simulink model "aircraft_arch"  (R2024a)
settings: Solver=FixedStepAuto  StartTime=0.0  StopTime=100.0  FixedStep=0.1  RelTol=1e-3
settings Model: Creator=amir  LastModifiedBy=amir
settings ConfigComp: CovEnable=on  RecordCoverage=on  CovEnableCumulative=off  CovModelRefEnable=on

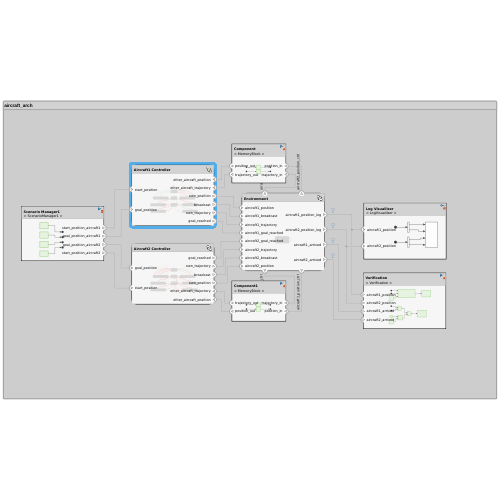
[thumbnail: Simulink's stored preview of the top-level diagram]
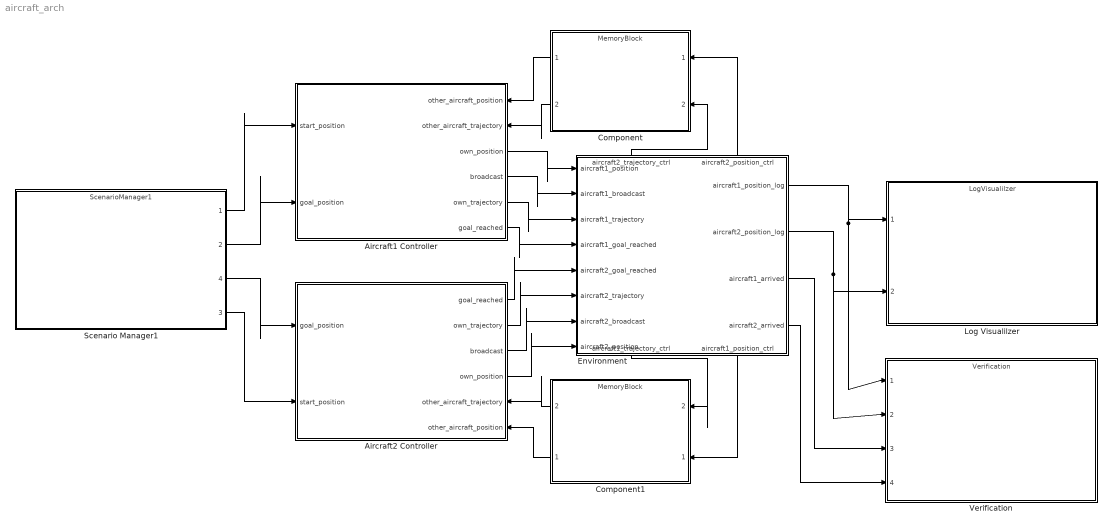
== system aircraft_arch ==
  Aircraft1 Controller : Stateflow chart  TreatAsAtomicUnit=on
      settings: PortSchema="{\"entries\":[{\"content\":{\"headerSize\":26,\"margin\":15,\"minimumSpacing\":25,\"sides\":[{\"content\":{\"connectorIds\":[\"In3\",\"In4\"]},\"type\":\"ConnectorPlacement.EquallySpacedRectSide\",\"uuid\":\"1f55804f-7089-4bd3-b638-e4b9c8b42ca4\"},{\"content\":{\"connectorIds\":[\"In1\",\"In2\",\"Out1\",\"Out2\",\"Out3\",\"Out4\"],\"side\":\"RIGHT\"},\"type\":\"ConnectorPlacement.EquallySpacedRectSide\",\"uuid\":\"b3c2471c-8380-46f0-98ab-243070185840\"},{\"content\":{\"side\":\"TOP\"},\"type\":\"ConnectorPlacement.EquallySpacedRectSide\",\"uuid\":\"f84a374d-020b-4849-aef2-6fb46c6d88bf\"}]},\"type\":\"ConnectorPlacement.EquallySpacedConnector\",\"uuid\":\"5317393d-ba95-4fee-8ac3-0dbadcfc5ad7\"}],\"packageUris\":[\"http://schema.mathworks.com/mf0/Connector/R2020b\"],\"version\":\"1.0\"}"
  Aircraft2 Controller : Stateflow chart  TreatAsAtomicUnit=on
      settings: PortSchema="{\"entries\":[{\"content\":{\"headerSize\":26,\"margin\":15,\"minimumSpacing\":25,\"sides\":[{\"content\":{\"connectorIds\":[\"In4\",\"In3\"]},\"type\":\"ConnectorPlacement.EquallySpacedRectSide\",\"uuid\":\"1f55804f-7089-4bd3-b638-e4b9c8b42ca4\"},{\"content\":{\"connectorIds\":[\"Out4\",\"Out3\",\"Out2\",\"Out1\",\"In1\",\"In2\"],\"side\":\"RIGHT\"},\"type\":\"ConnectorPlacement.EquallySpacedRectSide\",\"uuid\":\"b3c2471c-8380-46f0-98ab-243070185840\"},{\"content\":{\"side\":\"TOP\"},\"type\":\"ConnectorPlacement.EquallySpacedRectSide\",\"uuid\":\"f84a374d-020b-4849-aef2-6fb46c6d88bf\"}]},\"type\":\"ConnectorPlacement.EquallySpacedConnector\",\"uuid\":\"5317393d-ba95-4fee-8ac3-0dbadcfc5ad7\"}],\"packageUris\":[\"http://schema.mathworks.com/mf0/Connector/R2020b\"],\"version\":\"1.0\"}"
  Component : ModelReference  ModelNameDialog=MemoryBlock.slx  SimulationMode=Normal  ModelReferenceVersion=1.4
      settings: PortSchema="{\"entries\":[{\"content\":{\"headerSize\":38,\"margin\":15,\"minimumSpacing\":25,\"sides\":[{\"content\":{\"connectorIds\":[\"Out1\",\"Out2\"]},\"type\":\"ConnectorPlacement.EquallySpacedRectSide\",\"uuid\":\"1f55804f-7089-4bd3-b638-e4b9c8b42ca4\"},{\"content\":{\"connectorIds\":[\"In1\",\"In2\"],\"side\":\"RIGHT\"},\"type\":\"ConnectorPlacement.EquallySpacedRectSide\",\"uuid\":\"b3c2471c-8380-46f0-98ab-243070185840\"},{\"content\":{\"side\":\"TOP\"},\"type\":\"ConnectorPlacement.EquallySpacedRectSide\",\"uuid\":\"f84a374d-020b-4849-aef2-6fb46c6d88bf\"},{\"content\":{\"side\":\"BOTTOM\"},\"type\":\"ConnectorPlacement.EquallySpacedRectSide\",\"uuid\":\"1d177eb2-3e23-41ae-8748-2ec0886adf75\"}]},\"type\":\"ConnectorPlacement.EquallySpacedConnector\",\"uuid\":\"5317393d-ba95-4fee-8ac3-0dbadcfc5ad7\"}],\"packageUris\":[\"http://schema.mathworks.com/mf0/Connector/R2020b\"],\"version\":\"1.0\"}"
  Component1 : ModelReference  ModelNameDialog=MemoryBlock  SimulationMode=Normal  ModelReferenceVersion=1.4
      settings: PortSchema="{\"entries\":[{\"content\":{\"headerSize\":38,\"margin\":15,\"minimumSpacing\":25,\"sides\":[{\"content\":{\"connectorIds\":[\"Out2\",\"Out1\"]},\"type\":\"ConnectorPlacement.EquallySpacedRectSide\",\"uuid\":\"1f55804f-7089-4bd3-b638-e4b9c8b42ca4\"},{\"content\":{\"connectorIds\":[\"In2\",\"In1\"],\"side\":\"RIGHT\"},\"type\":\"ConnectorPlacement.EquallySpacedRectSide\",\"uuid\":\"b3c2471c-8380-46f0-98ab-243070185840\"},{\"content\":{\"side\":\"TOP\"},\"type\":\"ConnectorPlacement.EquallySpacedRectSide\",\"uuid\":\"f84a374d-020b-4849-aef2-6fb46c6d88bf\"},{\"content\":{\"side\":\"BOTTOM\"},\"type\":\"ConnectorPlacement.EquallySpacedRectSide\",\"uuid\":\"1d177eb2-3e23-41ae-8748-2ec0886adf75\"}]},\"type\":\"ConnectorPlacement.EquallySpacedConnector\",\"uuid\":\"5317393d-ba95-4fee-8ac3-0dbadcfc5ad7\"}],\"packageUris\":[\"http://schema.mathworks.com/mf0/Connector/R2020b\"],\"version\":\"1.0\"}"
  Environment : Stateflow chart  TreatAsAtomicUnit=on
      settings: PortSchema="{\"entries\":[{\"content\":{\"headerSize\":26,\"margin\":15,\"minimumSpacing\":25,\"sides\":[{\"content\":{\"connectorIds\":[\"In1\",\"In2\",\"In3\",\"In4\",\"In5\",\"In6\",\"In7\",\"In8\"]},\"type\":\"ConnectorPlacement.EquallySpacedRectSide\",\"uuid\":\"1f55804f-7089-4bd3-b638-e4b9c8b42ca4\"},{\"content\":{\"connectorIds\":[\"Out1\",\"Out4\",\"Out7\",\"Out8\"],\"side\":\"RIGHT\"},\"type\":\"ConnectorPlacement.EquallySpacedRectSide\",\"uuid\":\"b3c2471c-8380-46f0-98ab-243070185840\"},{\"content\":{\"connectorIds\":[\"Out3\",\"Out5\"],\"side\":\"TOP\"},\"type\":\"ConnectorPlacement.EquallySpacedRectSide\",\"uuid\":\"f84a374d-020b-4849-aef2-6fb46c6d88bf\"},{\"content\":{\"connectorIds\":[\"Out2\",\"Out6\"],\"side\":\"BOTTOM\"},\"type\":\"ConnectorPlacement.EquallySpacedRectSide\",\"uuid\":\"852cc804-b545-4d00-b17f-3ae2fc6b003e\"}]},\"type\":\"ConnectorPlacement.EquallySpacedConnector\",\"uuid\":\"5317393d-ba95-4fee-8ac3-0dbadcfc5ad7\"}],\"packageUris\":[\"http://schema.mathworks.com/mf0/Connector/R2020b\"],\"version\":\"1.0\"}"
  Log Visualilzer : ModelReference  ModelNameDialog=LogVisualilzer  SimulationMode=Normal  ModelReferenceVersion=1.7
      settings: PortSchema="{\"entries\":[{\"content\":{\"headerSize\":38,\"margin\":15,\"minimumSpacing\":25,\"sides\":[{\"content\":{\"connectorIds\":[\"In1\",\"In2\"]},\"type\":\"ConnectorPlacement.EquallySpacedRectSide\",\"uuid\":\"1f55804f-7089-4bd3-b638-e4b9c8b42ca4\"},{\"content\":{\"side\":\"RIGHT\"},\"type\":\"ConnectorPlacement.EquallySpacedRectSide\",\"uuid\":\"b3c2471c-8380-46f0-98ab-243070185840\"},{\"content\":{\"side\":\"TOP\"},\"type\":\"ConnectorPlacement.EquallySpacedRectSide\",\"uuid\":\"f84a374d-020b-4849-aef2-6fb46c6d88bf\"}]},\"type\":\"ConnectorPlacement.EquallySpacedConnector\",\"uuid\":\"5317393d-ba95-4fee-8ac3-0dbadcfc5ad7\"}],\"packageUris\":[\"http://schema.mathworks.com/mf0/Connector/R2020b\"],\"version\":\"1.0\"}"
  Scenario Manager1 : ModelReference  ModelNameDialog=ScenarioManager1.slx  SimulationMode=Normal  ModelReferenceVersion=1.20
      settings: PortSchema="{\"entries\":[{\"content\":{\"headerSize\":38,\"margin\":15,\"minimumSpacing\":25,\"sides\":[{\"content\":{},\"type\":\"ConnectorPlacement.EquallySpacedRectSide\",\"uuid\":\"1f55804f-7089-4bd3-b638-e4b9c8b42ca4\"},{\"content\":{\"connectorIds\":[\"Out1\",\"Out2\",\"Out4\",\"Out3\"],\"side\":\"RIGHT\"},\"type\":\"ConnectorPlacement.EquallySpacedRectSide\",\"uuid\":\"b3c2471c-8380-46f0-98ab-243070185840\"},{\"content\":{\"side\":\"TOP\"},\"type\":\"ConnectorPlacement.EquallySpacedRectSide\",\"uuid\":\"f84a374d-020b-4849-aef2-6fb46c6d88bf\"}]},\"type\":\"ConnectorPlacement.EquallySpacedConnector\",\"uuid\":\"5317393d-ba95-4fee-8ac3-0dbadcfc5ad7\"}],\"packageUris\":[\"http://schema.mathworks.com/mf0/Connector/R2020b\"],\"version\":\"1.0\"}"
  Verification : ModelReference  ModelNameDialog=Verification  SimulationMode=Normal  ModelReferenceVersion=1.8
      settings: PortSchema="{\"entries\":[{\"content\":{\"headerSize\":38,\"margin\":15,\"minimumSpacing\":25,\"sides\":[{\"content\":{\"connectorIds\":[\"In1\",\"In2\",\"In3\",\"In4\"]},\"type\":\"ConnectorPlacement.EquallySpacedRectSide\",\"uuid\":\"10c170e3-5d79-4eda-90c6-d87a95188a44\"},{\"content\":{\"side\":\"RIGHT\"},\"type\":\"ConnectorPlacement.EquallySpacedRectSide\",\"uuid\":\"ea2fd0a6-7ce8-495f-a83e-fe6cf76b2057\"},{\"content\":{\"side\":\"TOP\"},\"type\":\"ConnectorPlacement.EquallySpacedRectSide\",\"uuid\":\"87f50319-688b-4f7c-b51e-7381fe44f37b\"}]},\"type\":\"ConnectorPlacement.EquallySpacedConnector\",\"uuid\":\"e134149c-ef09-4213-a414-03764e4b3756\"}],\"packageUris\":[\"http://schema.mathworks.com/mf0/Connector/R2020b\"],\"version\":\"1.0\"}"
  wires:
  Scenario Manager1/2 -> Aircraft1 Controller/4(goal_position)
  Scenario Manager1/1 -> Aircraft1 Controller/3(start_position)
  Scenario Manager1/4 -> Aircraft2 Controller/4(goal_position)
  Scenario Manager1/3 -> Aircraft2 Controller/3(start_position)
  Aircraft1 Controller/1(own_position) -> Environment/1(aircraft1_position)
  Aircraft2 Controller/1(own_position) -> Environment/8(aircraft2_position)
  Aircraft2 Controller/2(broadcast) -> Environment/7(aircraft2_broadcast)
  Aircraft1 Controller/2(broadcast) -> Environment/2(aircraft1_broadcast)
  Environment/5(aircraft2_position_ctrl) -> Component/1
  Component/1 -> Aircraft1 Controller/1(other_aircraft_position)
  Component1/1 -> Aircraft2 Controller/2(other_aircraft_position)
  Aircraft1 Controller/3(own_trajectory) -> Environment/3(aircraft1_trajectory)
  Aircraft1 Controller/4(goal_reached) -> Environment/4(aircraft1_goal_reached)
  Environment/6(aircraft1_position_ctrl) -> Component1/1
  Aircraft2 Controller/3(own_trajectory) -> Environment/6(aircraft2_trajectory)
  Aircraft2 Controller/4(goal_reached) -> Environment/5(aircraft2_goal_reached)
  Environment/3(aircraft2_trajectory_ctrl) -> Component/2
  Component/2 -> Aircraft1 Controller/2(other_aircraft_trajectory)
  Environment/2(aircraft1_trajectory_ctrl) -> Component1/2
  Component1/2 -> Aircraft2 Controller/1(other_aircraft_trajectory)
  Environment/7(aircraft1_arrived) -> Verification/3
  Environment/1(aircraft1_position_log) -> Log Visualilzer/1, Verification/1
  Environment/8(aircraft2_arrived) -> Verification/4
  Environment/4(aircraft2_position_log) -> Log Visualilzer/2, Verification/2

== stateflow chart aircraft_arch/Aircraft2 Controller ==
  settings: updateMethod=CONTINUOUS
  state Idle
    during:
    own_position_dot(1) = 0;
    own_position_dot(2) = 0;
    broadcast = true;
  state CombsDelay
    during:
    own_position_dot(1) = 0;
    own_position_dot(2) = 0;
    broadcast = false;
  state VerticalMovement
    during:
    own_position_dot(2) = sign(goal_position(2) - own_position(2));
  state HorizontalMovement
    during:
    own_position_dot(1) = sign(goal_position(1) - own_position(1));
  state CorrectionManager
    during:
    own_position_dot(1) = 0;
    own_position_dot(2) = 0;
    broadcast = true;
  state HorizontalHeadOn_Side_CollisionAvoidance_VerticalMovement
    during:
    own_position_dot(1) = own_trajectory(2);
    own_position_dot(2) = -own_trajectory(1);
  state VerticalHeadOn_CollisionAvoidance_HorizontalMovement
    during:
    own_position_dot(1) = own_trajectory(2);
    own_position_dot(2) = -own_trajectory(1);
  state VerticalHeadOnCollisionAvoidanc_VerticalMovement
    during:
    own_position_dot(1) = own_trajectory(1);
    own_position_dot(2) = own_trajectory(2);
  state HeadButt_CollisionAvoidance
    during:
    own_position_dot(1) = -other_aircraft_trajectory(1);
    own_position_dot(2) = -other_aircraft_trajectory(2);
  (default) -> Idle : {own_position = start_position;
      | broadcast = true;
      | own_trajectory = [0, 0];
      | head_on_correction_step = 0;
      | vertical_trajectory=false;}
  VerticalMovement -> Idle [order 1] : [(abs(own_position(2) - round(own_position(2))) <= 0.01) && (abs(own_position(1) - goal_position(1)) > 0.01)]
      | {own_trajectory(1) = sign(goal_position(1) - own_position(1)); own_trajectory(2) = 0; vertical_trajectory = false;}
  HorizontalMovement -> Idle [order 1] : [(abs(own_position(1) - round(own_position(1))) <= 0.01) && (abs(own_position(1) - goal_position(1)) > 0.01)]
      | {own_trajectory(1) = sign(goal_position(1) - own_position(1)); own_trajectory(2) = 0;}
  HorizontalMovement -> Idle [order 2] : [(abs(own_position(1) - round(own_position(1))) <= 0.01) && (abs(own_position(2) - goal_position(2)) > 0.01)]
      | {own_trajectory(1) = 0; own_trajectory(2) = sign(goal_position(2) - own_position(2));}
  VerticalMovement -> Idle [order 2] : [(abs(own_position(2) - round(own_position(2))) <= 0.01) && (abs(own_position(2) - goal_position(2)) > 0.01)]
      | {own_trajectory(1) = 0; own_trajectory(2) = sign(goal_position(2) - own_position(2)); vertical_trajectory = false;}
  VerticalMovement -> Idle [order 3] : [(abs(own_position(1) - round(own_position(1))) <= 0.01) && (abs(own_position(2) - round(own_position(2))) <= 0.01)]
      | {goal_reached = true; vertical_trajectory = false;}
  HorizontalMovement -> Idle [order 3] : [(abs(own_position(1) - round(own_position(1))) <= 0.01) && (abs(own_position(2) - round(own_position(2))) <= 0.01)]
      | {goal_reached = true;}
  Idle -> CombsDelay : [(abs(own_position(1) - goal_position(1)) > 0.01) || (abs(own_position(2) - goal_position(2)) > 0.01)]
  CombsDelay -> HorizontalMovement [order 4] : [(abs(own_position(1) - goal_position(1)) > 0.01) && ~vertical_trajectory]
  CombsDelay -> VerticalMovement [order 5] : [(abs(own_position(2) - goal_position(2)) > 0.01) || vertical_trajectory]
  CombsDelay -> (junction 360) [order 1] : [(all(round(own_position) + own_trajectory == round(other_aircraft_position) + other_aircraft_trajectory) || ...
      |  all(round(own_position) + 0.5 * own_trajectory == round(other_aircraft_position) + 0.5 * other_aircraft_trajectory)) && ...
      |  (all(abs(round(own_trajectory - other_aircraft_trajectory)) == [2, 0]) || ...
      |  all(abs(round(own_trajectory - other_aircraft_trajectory)) == [1, 1]))]
  CombsDelay -> VerticalHeadOn_CollisionAvoidance_HorizontalMovement [order 2] : [(all(round(own_position) + own_trajectory == round(other_aircraft_position) + other_aircraft_trajectory) || ...
      |  all(round(own_position) + 0.5 * own_trajectory == round(other_aircraft_position) + 0.5 * other_aircraft_trajectory)) && ...
      |  all(abs(round(own_trajectory - other_aircraft_trajectory)) == [0, 2])]
      | {head_on_correction_step = abs(round(own_position(2)) - round(other_aircraft_position(2)));}
  CorrectionManager -> CombsDelay [order 2]
  CombsDelay -> (junction 351) [order 3] : [all(round(own_position) + own_trajectory == round(other_aircraft_position))]
  (junction 360) -> HorizontalHeadOn_Side_CollisionAvoidance_VerticalMovement [order 1] : [abs(round(own_trajectory)) == [0, 1]]
      | {vertical_trajectory = true;}
  (junction 360) -> HorizontalHeadOn_Side_CollisionAvoidance_VerticalMovement [order 2]
  VerticalHeadOn_CollisionAvoidance_HorizontalMovement -> CorrectionManager : [(abs(own_position(1) - round(own_position(1))) <= 0.01)]
  HorizontalHeadOn_Side_CollisionAvoidance_VerticalMovement -> CorrectionManager : [(~vertical_trajectory && abs(own_position(2) - round(own_position(2))) <= 0.01) || ...
      |  (vertical_trajectory && abs(own_position(1) - round(own_position(1))) <= 0.01)]
  CorrectionManager -> VerticalHeadOnCollisionAvoidanc_VerticalMovement [order 1] : [head_on_correction_step ~= 0]
  VerticalHeadOnCollisionAvoidanc_VerticalMovement -> CorrectionManager : [(abs(own_position(2) - round(own_position(2))) <= 0.01)]
      | {head_on_correction_step = head_on_correction_step - 1}
  HeadButt_CollisionAvoidance -> CorrectionManager : [(~vertical_trajectory && abs(own_position(2) - round(own_position(2))) <= 0.01) || ...
      |  (vertical_trajectory && abs(own_position(1) - round(own_position(1))) <= 0.01)]
  (junction 351) -> HeadButt_CollisionAvoidance [order 1] : [abs(round(own_trajectory)) == [0, 1]]
      | {vertical_trajectory = true;}
  (junction 351) -> HeadButt_CollisionAvoidance [order 2]
  data: other_aircraft_trajectory input size=[1, 2]; other_aircraft_position input size=[1, 2]; start_position input size=[1, 2]; goal_position input size=[1, 2]; own_position output size=[1, 2]; broadcast output boolean; own_trajectory output size=[1, 2]; goal_reached output boolean; head_on_correction_step local; vertical_trajectory local boolean
  data own_position settings: updateMethod=SF_CONTINUOUS_TIME_DATA
  data own_trajectory settings: updateMethod=SF_CONTINUOUS_TIME_DATA

== stateflow chart aircraft_arch/Environment ==
  settings: updateMethod=CONTINUOUS
  state LogPass
    during:
    aircraft1_position_log = aircraft1_position;
    aircraft2_position_log = aircraft2_position;
    aircraft1_arrived = aircraft1_goal_reached;
    aircraft2_arrived = aircraft2_goal_reached;
  (default) -> LogPass : {aircraft1_position_log = aircraft1_position;
      | aircraft1_position_ctrl = [10000, 10000];
      | aircraft1_trajectory_ctrl = [0, 0];
      | aircraft2_position_log = aircraft2_position;
      | aircraft2_position_ctrl = [10000, 10000];
      | aircraft2_trajectory_ctrl = [0, 0];}
  LogPass -> LogPass [order 2] : [aircraft1_broadcast && aircraft2_broadcast && ...
      |  (aircraft1_goal_reached || aircraft2_goal_reached || ...
      |   (abs(round(aircraft1_position(1)) - round(aircraft2_position(1))) > 2) || ...
      |   (abs(round(aircraft1_position(2)) - round(aircraft2_position(2))) > 2))]
      | {aircraft1_position_ctrl   = [10000, 10000];
      |  aircraft1_trajectory_ctrl = [0, 0];
      |  aircraft2_position_ctrl   = [10000, 10000];
      |  aircraft2_trajectory_ctrl = [0, 0];}
  LogPass -> LogPass [order 1] : [aircraft1_broadcast && aircraft2_broadcast && ...
      |  ~aircraft1_goal_reached && ~aircraft2_goal_reached && ...
      |  (abs(round(aircraft1_position(1)) - round(aircraft2_position(1))) <= 2) && ...
      |  (abs(round(aircraft1_position(2)) - round(aircraft2_position(2))) <= 2)]
      | {aircraft1_position_log = aircraft1_position;
      |  aircraft1_position_ctrl = aircraft1_position;
      |  aircraft1_trajectory_ctrl = aircraft1_trajectory;
      |  aircraft2_position_log = aircraft2_position;
      |  aircraft2_position_ctrl = aircraft2_position;
      |  aircraft2_trajectory_ctrl = aircraft2_trajectory;}
  data: aircraft1_position input size=[1, 2]; aircraft1_broadcast input boolean; aircraft1_trajectory input size=[1, 2]; aircraft1_goal_reached input boolean; aircraft2_goal_reached input boolean; aircraft2_trajectory input size=[1, 2]; aircraft2_broadcast input boolean; aircraft2_position input size=[1, 2]; aircraft1_position_log output size=[1, 2]; aircraft1_trajectory_ctrl output; aircraft2_trajectory_ctrl output; aircraft2_position_log output size=[1, 2]; aircraft2_position_ctrl output size=[1, 2]; aircraft1_position_ctrl output size=[1, 2]; aircraft1_arrived output boolean; aircraft2_arrived output boolean

== stateflow chart aircraft_arch/Aircraft1 Controller ==
  settings: updateMethod=CONTINUOUS
  state Idle
    during:
    own_position_dot(1) = 0;
    own_position_dot(2) = 0;
    broadcast = true;
  state CombsDelay
    during:
    own_position_dot(1) = 0;
    own_position_dot(2) = 0;
    broadcast = false;
  state VerticalMovement
    during:
    own_position_dot(2) = sign(goal_position(2) - own_position(2));
  state HorizontalMovement
    during:
    own_position_dot(1) = sign(goal_position(1) - own_position(1));
  state CorrectionManager
    during:
    own_position_dot(1) = 0;
    own_position_dot(2) = 0;
    broadcast = true;
  state HorizontalHeadOn_Side_CollisionAvoidance_VerticalMovement
    during:
    own_position_dot(1) = own_trajectory(2);
    own_position_dot(2) = -own_trajectory(1);
  state VerticalHeadOn_CollisionAvoidance_HorizontalMovement
    during:
    own_position_dot(1) = own_trajectory(2);
    own_position_dot(2) = -own_trajectory(1);
  state VerticalHeadOnCollisionAvoidanc_VerticalMovement
    during:
    own_position_dot(1) = own_trajectory(1);
    own_position_dot(2) = own_trajectory(2);
  state HeadButt_CollisionAvoidance
    during:
    own_position_dot(1) = -other_aircraft_trajectory(1);
    own_position_dot(2) = -other_aircraft_trajectory(2);
  (default) -> Idle : {own_position = start_position;
      | broadcast = true;
      | own_trajectory = [0, 0];
      | head_on_correction_step = 0;
      | vertical_trajectory=false;}
  VerticalMovement -> Idle [order 1] : [(abs(own_position(2) - round(own_position(2))) <= 0.01) && (abs(own_position(1) - goal_position(1)) > 0.01)]
      | {own_trajectory(1) = sign(goal_position(1) - own_position(1)); own_trajectory(2) = 0; vertical_trajectory = false;}
  HorizontalMovement -> Idle [order 1] : [(abs(own_position(1) - round(own_position(1))) <= 0.01) && (abs(own_position(1) - goal_position(1)) > 0.01)]
      | {own_trajectory(1) = sign(goal_position(1) - own_position(1)); own_trajectory(2) = 0;}
  HorizontalMovement -> Idle [order 2] : [(abs(own_position(1) - round(own_position(1))) <= 0.01) && (abs(own_position(2) - goal_position(2)) > 0.01)]
      | {own_trajectory(1) = 0; own_trajectory(2) = sign(goal_position(2) - own_position(2));}
  VerticalMovement -> Idle [order 2] : [(abs(own_position(2) - round(own_position(2))) <= 0.01) && (abs(own_position(2) - goal_position(2)) > 0.01)]
      | {own_trajectory(1) = 0; own_trajectory(2) = sign(goal_position(2) - own_position(2)); vertical_trajectory = false;}
  VerticalMovement -> Idle [order 3] : [(abs(own_position(1) - round(own_position(1))) <= 0.01) && (abs(own_position(2) - round(own_position(2))) <= 0.01)]
      | {goal_reached = true; vertical_trajectory = false;}
  HorizontalMovement -> Idle [order 3] : [(abs(own_position(1) - round(own_position(1))) <= 0.01) && (abs(own_position(2) - round(own_position(2))) <= 0.01)]
      | {goal_reached = true;}
  Idle -> CombsDelay : [(abs(own_position(1) - goal_position(1)) > 0.01) || (abs(own_position(2) - goal_position(2)) > 0.01)]
  CombsDelay -> HorizontalMovement [order 4] : [(abs(own_position(1) - goal_position(1)) > 0.01) && ~vertical_trajectory]
  CombsDelay -> VerticalMovement [order 5] : [(abs(own_position(2) - goal_position(2)) > 0.01) || vertical_trajectory]
  CombsDelay -> (junction 99) [order 1] : [(all(round(own_position) + own_trajectory == round(other_aircraft_position) + other_aircraft_trajectory) || ...
      |  all(round(own_position) + 0.5 * own_trajectory == round(other_aircraft_position) + 0.5 * other_aircraft_trajectory)) && ...
      |  (all(abs(round(own_trajectory - other_aircraft_trajectory)) == [2, 0]) || ...
      |  all(abs(round(own_trajectory - other_aircraft_trajectory)) == [1, 1]))]
  CombsDelay -> VerticalHeadOn_CollisionAvoidance_HorizontalMovement [order 2] : [(all(round(own_position) + own_trajectory == round(other_aircraft_position) + other_aircraft_trajectory) || ...
      |  all(round(own_position) + 0.5 * own_trajectory == round(other_aircraft_position) + 0.5 * other_aircraft_trajectory)) && ...
      |  all(abs(round(own_trajectory - other_aircraft_trajectory)) == [0, 2])]
      | {head_on_correction_step = abs(round(own_position(2)) - round(other_aircraft_position(2)));}
  CorrectionManager -> CombsDelay [order 2]
  CombsDelay -> (junction 125) [order 3] : [all(round(own_position) + own_trajectory == round(other_aircraft_position))]
  (junction 99) -> HorizontalHeadOn_Side_CollisionAvoidance_VerticalMovement [order 1] : [abs(round(own_trajectory)) == [0, 1]]
      | {vertical_trajectory = true;}
  (junction 99) -> HorizontalHeadOn_Side_CollisionAvoidance_VerticalMovement [order 2]
  VerticalHeadOn_CollisionAvoidance_HorizontalMovement -> CorrectionManager : [(abs(own_position(1) - round(own_position(1))) <= 0.01)]
  HorizontalHeadOn_Side_CollisionAvoidance_VerticalMovement -> CorrectionManager : [(~vertical_trajectory && abs(own_position(2) - round(own_position(2))) <= 0.01) || ...
      |  (vertical_trajectory && abs(own_position(1) - round(own_position(1))) <= 0.01)]
  CorrectionManager -> VerticalHeadOnCollisionAvoidanc_VerticalMovement [order 1] : [head_on_correction_step ~= 0]
  VerticalHeadOnCollisionAvoidanc_VerticalMovement -> CorrectionManager : [(abs(own_position(2) - round(own_position(2))) <= 0.01)]
      | {head_on_correction_step = head_on_correction_step - 1}
  HeadButt_CollisionAvoidance -> CorrectionManager : [(~vertical_trajectory && abs(own_position(2) - round(own_position(2))) <= 0.01) || ...
      |  (vertical_trajectory && abs(own_position(1) - round(own_position(1))) <= 0.01)]
  (junction 125) -> HeadButt_CollisionAvoidance [order 1] : [abs(round(own_trajectory)) == [0, 1]]
      | {vertical_trajectory = true;}
  (junction 125) -> HeadButt_CollisionAvoidance [order 2]
  data: other_aircraft_position input size=[1, 2]; other_aircraft_trajectory input size=[1, 2]; start_position input size=[1, 2]; goal_position input size=[1, 2]; own_position output size=[1, 2]; broadcast output boolean; own_trajectory output size=[1, 2]; goal_reached output boolean; head_on_correction_step local; vertical_trajectory local boolean
  data own_position settings: updateMethod=SF_CONTINUOUS_TIME_DATA
  data own_trajectory settings: updateMethod=SF_CONTINUOUS_TIME_DATA
